simulink library "ddc_lib"  (R2022b)
settings: Solver=VariableStepAuto  StartTime=0.0  StopTime=10.0  RelTol=1e-3
settings Model: Creator=armangb1  LastModifiedBy=armangb1
settings OptimizationCC: ReuseModelBlockBuffer=on
settings RTWCC: GPUComputeCapability=5.0

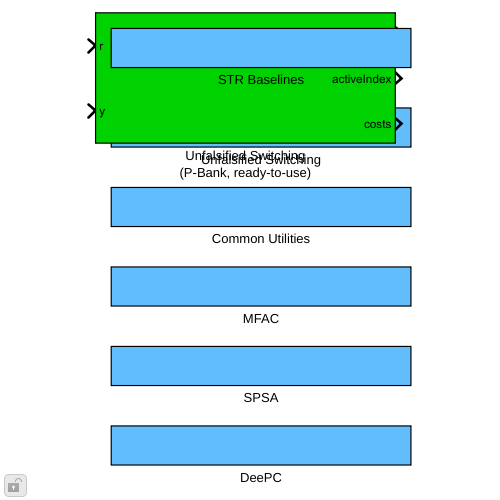
[thumbnail: Simulink's stored preview of the top-level diagram]
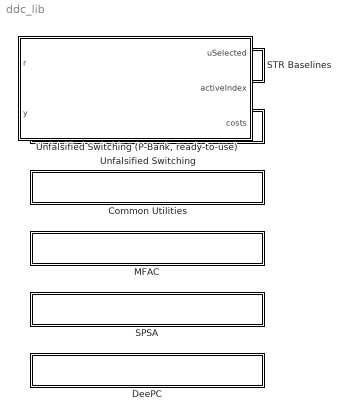
== system ddc_lib ==
  Common Utilities : Subsystem
  DeePC : Subsystem
  MFAC : Subsystem
  SPSA : Subsystem
  STR Baselines : Subsystem
  Unfalsified Switching : Subsystem
  "Unfalsified Switching (P-Bank, ready-to-use)" : Subsystem  mask(Unfalsified Switching (P-Bank)){Controllers=[0.5; 1; 2]}
      mask prompts: Controllers "Candidate controllers"
      mask help: Ready-to-use unfalsified adaptive switching control block: a bank of proportional candidate controllers plus the cost-based switching logic, pre-wired. Set Controllers to the candidate controllers as a tf array or a vector of proportional gains.

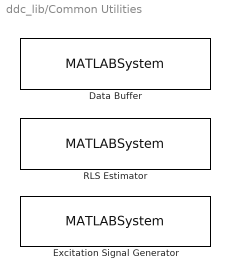
== system ddc_lib/Common Utilities ==
  Data Buffer : MATLABSystem  System=ddc.common.DataBuffer  WindowLength=10  SignalWidth=1  SimulateUsing=Code generation
      mask Type: ddc.common.DataBuffer
      mask Display:
      | disp('DataBuffer');
      | port_label('input',1,'sample');
      | port_label('output',1,'isFull');
      | port_label('output',2,'data');
  Excitation Signal Generator : MATLABSystem  System=ddc.common.ExcitationSignalGenerator  Amplitude=1  Seed=0  SwitchProbability=0.5  SimulateUsing=Code generation
      settings: SignalType=prbs
      mask Type: ddc.common.ExcitationSignalGenerator
      mask Display:
      | disp('ExcitationSignalGenerator');
      | port_label('output',1,'u');
  RLS Estimator : MATLABSystem  System=ddc.common.RLSEstimator  NumParameters=1  ExternalReset=off  ForgettingFactor=1  InitialCovarianceGain=10000  SimulateUsing=Code generation
      mask Type: ddc.common.RLSEstimator
      mask Display:
      | disp('RLSEstimator');
      | port_label('input',1,'phi');
      | port_label('input',2,'y');
      | port_label('output',1,'theta');
      | port_label('output',2,'predictionError');

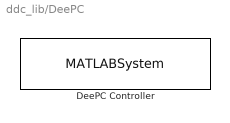
== system ddc_lib/DeePC ==
  DeePC Controller : MATLABSystem  System=ddc.deepc.DeePCController  DataU=[]  DataY=[]  Tini=4  N=10  AssumedOrder=0  SampleTime=-1  Q=1  R=0.01  LambdaG=1  LambdaY=10000  SimulateUsing=Code generation
      mask Type: ddc.deepc.DeePCController
      mask Display:
      | disp('DeePCController');
      | port_label('input',1,'yCurr');
      | port_label('input',2,'rFuture');
      | port_label('output',1,'uApply');
      | port_label('output',2,'yPred');

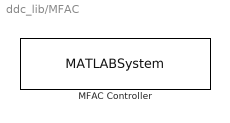
== system ddc_lib/MFAC ==
  MFAC Controller : MATLABSystem  System=ddc.mfac.MFACController  Ly=0  Lu=1  PhiInit=1  SampleTime=-1  Eta=1  Mu=1  Rho=1  Lambda=1  Epsilon=1e-05  SimulateUsing=Code generation
      mask Type: ddc.mfac.MFACController
      mask Display:
      | disp('MFACController');
      | port_label('input',1,'y');
      | port_label('input',2,'rNext');
      | port_label('output',1,'u');
      | port_label('output',2,'phiOut');

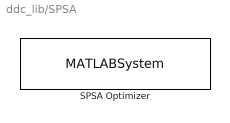
== system ddc_lib/SPSA ==
  SPSA Optimizer : MATLABSystem  System=ddc.spsa.SPSAOptimizer  NumParameters=1  InitialTheta=0  ParameterUpdateMode=immediate  SampleTime=-1  ATuning=0.1  CTuning=0.1  ACommon=10  Alpha=0.602  Gamma=0.101  SimulateUsing=Code generation
      mask Type: ddc.spsa.SPSAOptimizer
      mask Display:
      | disp('SPSAOptimizer');
      | port_label('input',1,'lossMeasurement');
      | port_label('output',1,'paramToApply');
      | port_label('output',2,'thetaEstimate');

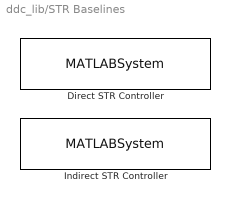
== system ddc_lib/STR Baselines ==
  Direct STR Controller : MATLABSystem  System=ddc.str.DirectSTRController  SampleTime=-1  Ac1=-0.5  ForgettingFactor=0.98  MinBeta0=0.001  InitialS0=0  InitialT0=1  SimulateUsing=Code generation
      mask Type: ddc.str.DirectSTRController
      mask Display:
      | disp('DirectSTRController');
      | port_label('input',1,'y');
      | port_label('input',2,'r');
      | port_label('output',1,'u');
      | port_label('output',2,'theta');
  Indirect STR Controller : MATLABSystem  System=ddc.str.IndirectSTRController  Na=1  Nb=1  SampleTime=-1  Am=[1 -0.5]  Bm=0.5  ObserverPole=0  ForgettingFactor=0.98  MinB=0.001  SimulateUsing=Code generation
      mask Type: ddc.str.IndirectSTRController
      mask Display:
      | disp('IndirectSTRController');
      | port_label('input',1,'y');
      | port_label('input',2,'r');
      | port_label('output',1,'u');
      | port_label('output',2,'theta');

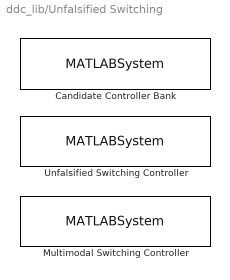
== system ddc_lib/Unfalsified Switching ==
  Candidate Controller Bank : MATLABSystem  System=ddc.ufc.CandidateControllerBank  Controllers=tf  SampleTime=-1  DiscretizationMethod=zoh  SimulateUsing=Code generation
      mask Type: ddc.ufc.CandidateControllerBank
      mask Display:
      | disp('CandidateControllerBank');
      | port_label('input',1,'r');
      | port_label('input',2,'y');
      | port_label('output',1,'uCandidates');
  Multimodal Switching Controller : MATLABSystem  System=ddc.ufc.MultimodelSwitchingController  Controllers=tf  Models=tf  SampleTime=-1  DiscretizationMethod=zoh  ForgettingFactor=0.95  HysteresisMargin=0.001  Epsilon=1e-12  SimulateUsing=Code generation
      mask Type: ddc.ufc.MultimodelSwitchingController
      mask Display:
      | disp('MultimodelSwitchingController');
      | port_label('input',1,'uCandidates');
      | port_label('input',2,'y');
      | port_label('output',1,'uSelected');
      | port_label('output',2,'activeIndex');
      | port_label('output',3,'costs');
  Unfalsified Switching Controller : MATLABSystem  System=ddc.ufc.UnfalsifiedSwitchingController  Controllers=tf  SampleTime=-1  DiscretizationMethod=zoh  ForgettingFactor=0.95  HysteresisMargin=0.001  Epsilon=1e-12  W1=1  W2=1  SimulateUsing=Code generation
      mask Type: ddc.ufc.UnfalsifiedSwitchingController
      mask Display:
      | disp('UnfalsifiedSwitchingController');
      | port_label('input',1,'uCandidates');
      | port_label('input',2,'y');
      | port_label('output',1,'uSelected');
      | port_label('output',2,'activeIndex');
      | port_label('output',3,'costs');

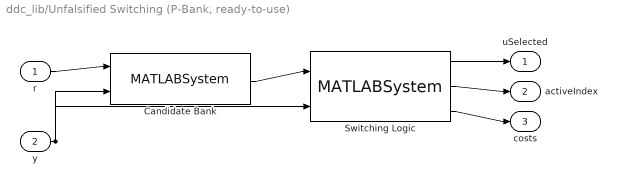
== system ddc_lib/Unfalsified Switching (P-Bank, ready-to-use) ==
  r : Inport
  y : Inport  Port=2
  Candidate Bank : MATLABSystem  System=ddc.ufc.CandidateControllerBank  Controllers=Controllers  SampleTime=-1  DiscretizationMethod=zoh  SimulateUsing=Code generation
      mask Type: ddc.ufc.CandidateControllerBank
      mask Display:
      | disp('CandidateControllerBank');
      | port_label('input',1,'r');
      | port_label('input',2,'y');
      | port_label('output',1,'uCandidates');
  Switching Logic : MATLABSystem  System=ddc.ufc.UnfalsifiedSwitchingController  Controllers=Controllers  SampleTime=-1  DiscretizationMethod=zoh  ForgettingFactor=0.95  HysteresisMargin=0.001  Epsilon=1e-12  W1=1  W2=1  SimulateUsing=Code generation
      mask Type: ddc.ufc.UnfalsifiedSwitchingController
      mask Display:
      | disp('UnfalsifiedSwitchingController');
      | port_label('input',1,'uCandidates');
      | port_label('input',2,'y');
      | port_label('output',1,'uSelected');
      | port_label('output',2,'activeIndex');
      | port_label('output',3,'costs');
  uSelected : Outport
  activeIndex : Outport  Port=2
  costs : Outport  Port=3
  wires:
  r/1 -> Candidate Bank/1
  y/1 -> Candidate Bank/2, Switching Logic/2
  Candidate Bank/1 -> Switching Logic/1
  Switching Logic/1 -> uSelected/1
  Switching Logic/2 -> activeIndex/1
  Switching Logic/3 -> costs/1
